simulink model "Fig1_4"  (R2019b)
settings: Solver=VariableStepAuto  StartTime=0.0  StopTime=10.0  RelTol=1e-3
PreLoadFcn:
  | R =1e2;
  | c =1e-2;
settings Model: Creator=Ommie  LastModifiedBy=Ommie

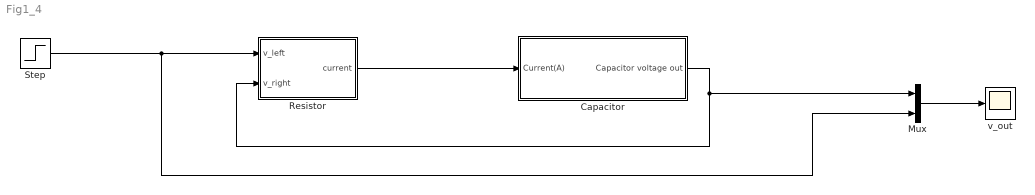
== system Fig1_4 ==
  "Capacitor " : Subsystem
  Mux : Mux  Inputs=2
  "Resistor " : Subsystem
  "Step " : Step  SampleTime=0
  v_out : Scope
  wires:
  "Step "/1 -> Mux/2, "Resistor "/1(v_left)
  "Capacitor "/1(Capacitor voltage out) -> Mux/1, "Resistor "/2(v_right)
  "Resistor "/1(current) -> "Capacitor "/1(Current(A))
  Mux/1 -> v_out/1

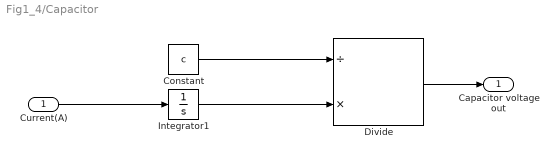
== system Fig1_4/Capacitor  ==
  Current(A) : Inport
  "Constant " : Constant  Value=c
  "Divide " : Product  Inputs=/*
  "Integrator1 " : Integrator
  Capacitor voltage out : Outport
  wires:
  "Constant "/1 -> "Divide "/1
  "Divide "/1 -> Capacitor voltage out/1
  "Integrator1 "/1 -> "Divide "/2
  Current(A)/1 -> "Integrator1 "/1

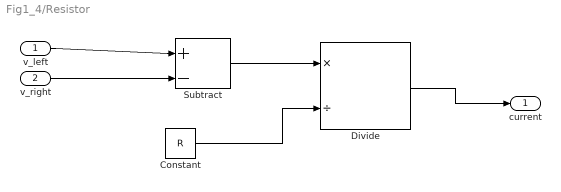
== system Fig1_4/Resistor  ==
  v_left : Inport
  v_right : Inport  Port=2
  "Constant " : Constant  Value=R
  "Divide " : Product  Inputs=*/
  "Subtract " : Sum  Inputs=+|-
  current : Outport
  wires:
  "Divide "/1 -> current/1
  "Constant "/1 -> "Divide "/2
  v_right/1 -> "Subtract "/2
  "Subtract "/1 -> "Divide "/1
  v_left/1 -> "Subtract "/1
